simulink model "validation_simulations_elena_P"  (R2019b)
settings: Solver=FixedStepAuto  StartTime=0.0  StopTime=20  FixedStep=0.002  RelTol=1e-3
undefined symbols (not defined in the file or in its folder): Ao, Bo, Co, kalmf, Klqi_int, Klqi_state, Kpp_int, Kpp_state, Parameters
settings Model: Creator=Samsung  LastModifiedBy=pietr

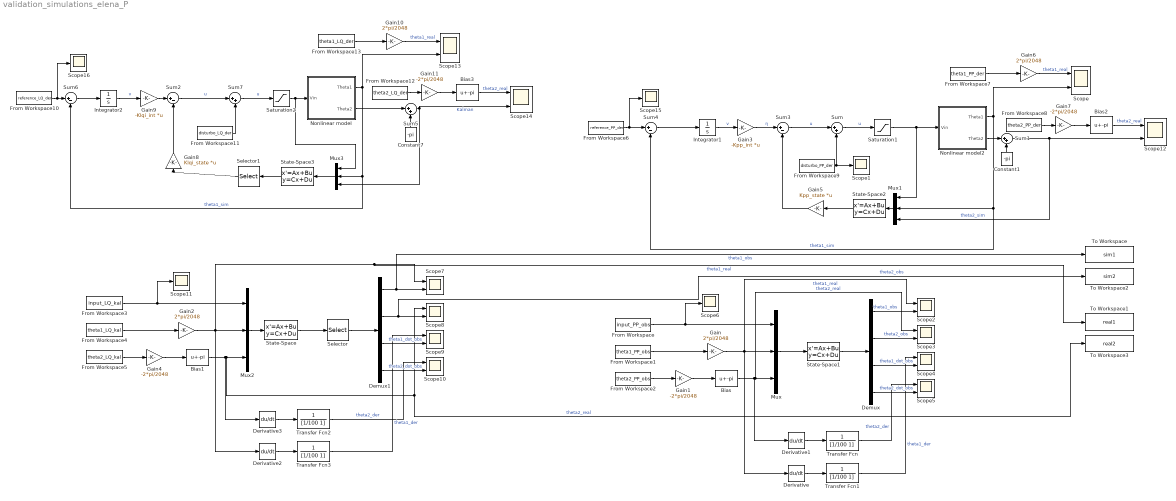
== system validation_simulations_elena_P ==
  Bias{,1..3} (4 alike) : Bias  Bias=-pi
  Constant1 : Constant  Value=-pi
  Constant7 : Constant  Value=-pi
  Demux : Demux
  Demux1 : Demux
  Derivative{,1..3} (4 alike) : Derivative
  From Workspace : FromWorkspace  VariableName=input_PP_obs  SampleTime=0
  From Workspace1 : FromWorkspace  VariableName=theta1_PP_obs  SampleTime=0
  From Workspace10 : FromWorkspace  VariableName=reference_LQ_der  SampleTime=0
  From Workspace11 : FromWorkspace  VariableName=disturbo_LQ_der  SampleTime=0
  From Workspace12 : FromWorkspace  VariableName=theta2_LQ_der  SampleTime=0
  From Workspace13 : FromWorkspace  VariableName=theta1_LQ_der  SampleTime=0
  From Workspace2 : FromWorkspace  VariableName=theta2_PP_obs  SampleTime=0
  From Workspace3 : FromWorkspace  VariableName=input_LQ_kal  SampleTime=0
  From Workspace4 : FromWorkspace  VariableName=theta1_LQ_kal  SampleTime=0
  From Workspace5 : FromWorkspace  VariableName=theta2_LQ_kal  SampleTime=0
  From Workspace6 : FromWorkspace  VariableName=reference_PP_der  SampleTime=0
  From Workspace7 : FromWorkspace  VariableName=theta1_PP_der  SampleTime=0
  From Workspace8 : FromWorkspace  VariableName=theta2_PP_der  SampleTime=0
  From Workspace9 : FromWorkspace  VariableName=disturbo_PP_der  SampleTime=0
  Gain{,2,6,10} (4 alike) : Gain  Gain=2*pi/2048
  Gain{1,4,7,11} (4 alike) : Gain  Gain=-2*pi/2048
  Gain3 : Gain  Gain=-Kpp_int  Multiplication=Matrix(K*u)
  Gain5 : Gain  Gain=Kpp_state  Multiplication=Matrix(K*u)
  Gain8 : Gain  Gain=Klqi_state  Multiplication=Matrix(K*u)
  Gain9 : Gain  Gain=-Klqi_int  Multiplication=Matrix(K*u)
  Integrator1 : Integrator
  Integrator2 : Integrator
  Mux{,1..3} (4 alike) : Mux  Inputs=3
  Nonlinear model : Subsystem
  Nonlinear model2 : Subsystem
  Saturation1 : Saturate  UpperLimit=10  LowerLimit=-10
  Saturation2 : Saturate  UpperLimit=10  LowerLimit=-10
  Scope{,2..5,7..10,12..14} (12 alike) : Scope  NumInputPorts=2
  Scope{1,6,11,15..16} (5 alike) : Scope
  Selector : Selector  InputPortWidth=6  IndexOptions=Index vector (dialog)  Indices=[3,4,5,6]  OutputSizes=1
  Selector1 : Selector  InputPortWidth=6  IndexOptions=Index vector (dialog)  Indices=[3,4,5,6]  OutputSizes=1
  State-Space : StateSpace  A=kalmf.A  B=kalmf.B  C=kalmf.C  D=kalmf.D  InitialCondition=[0,0,0,0]
  State-Space1 : StateSpace  A=Ao  B=Bo  C=Co  D=zeros(4,3)  InitialCondition=[0,0,0,0]
  State-Space2 : StateSpace  A=Ao  B=Bo  C=Co  D=zeros(4,3)  InitialCondition=[0,0,0,0]
  State-Space3 : StateSpace  A=kalmf.A  B=kalmf.B  C=kalmf.C  D=kalmf.D  InitialCondition=[0,0,0,0]
  Sum{,1,5,7} (4 alike) : Sum  Inputs=|++
  Sum{2..4,6} (4 alike) : Sum  Inputs=|+-
  To Workspace : ToWorkspace  VariableName=sim1  SampleTime=-1
      settings: Save2DSignal=2-D array (concatenate along first dimension)
  To Workspace1 : ToWorkspace  VariableName=real1  SampleTime=-1
      settings: Save2DSignal=2-D array (concatenate along first dimension)
  To Workspace2 : ToWorkspace  VariableName=sim2  SampleTime=-1
      settings: Save2DSignal=2-D array (concatenate along first dimension)
  To Workspace3 : ToWorkspace  VariableName=real2  SampleTime=-1
      settings: Save2DSignal=2-D array (concatenate along first dimension)
  Transfer Fcn{,1..3} (4 alike) : TransferFcn  Denominator=[1/100 1]
  wires:
  State-Space2/1 -> Gain5/1
  Sum4/1 -> Integrator1/1
  Nonlinear model2/2(Theta2) -> Sum1/1
  Gain5/1 -> Sum3/2
  Nonlinear model2/1(Theta1) -> Scope/2, Mux1/2, Sum4/2  "theta1_sim"
  Sum/1 -> Saturation1/1  "u"
  Constant1/1 -> Sum1/2
  Saturation1/1 -> Mux1/1, Nonlinear model2/1(Vin)
  Integrator1/1 -> Gain3/1  "v"
  Mux1/1 -> State-Space2/1
  Gain3/1 -> Sum3/1  "η"
  Sum1/1 -> Mux1/3, Scope12/2  "theta2_sim"
  Mux/1 -> State-Space1/1
  State-Space1/1 -> Demux/1
  Gain/1 -> Scope2/1, Derivative/1, Mux/2  "theta1_real"
  Gain1/1 -> Bias/1
  Demux/1 -> Scope2/2  "theta1_obs"
  Demux/2 -> Scope3/2  "theta2_obs"
  Demux/3 -> Scope4/2  "theta1_dot_obs"
  Demux/4 -> Scope5/2  "theta2_dot_obs"
  Derivative1/1 -> Transfer Fcn/1
  Derivative/1 -> Transfer Fcn1/1
  Transfer Fcn/1 -> Scope5/1  "theta2_der"
  Transfer Fcn1/1 -> Scope4/1  "theta1_der"
  From Workspace1/1 -> Gain/1
  From Workspace2/1 -> Gain1/1
  From Workspace/1 -> Scope6/1, Mux/1
  Bias/1 -> Scope3/1, Mux/3, Derivative1/1  "theta2_real"
  State-Space/1 -> Selector/1
  Mux2/1 -> State-Space/1
  From Workspace5/1 -> Gain4/1
  Transfer Fcn2/1 -> Scope10/1  "theta2_der"
  Demux1/1 -> To Workspace/1, Scope7/2  "theta1_obs"
  Bias1/1 -> Scope8/1, To Workspace3/1, Mux2/3, Derivative3/1  "theta2_real"
  From Workspace3/1 -> Scope11/1, Mux2/1
  Demux1/2 -> To Workspace2/1, Scope8/2  "theta2_obs"
  From Workspace4/1 -> Gain2/1
  Transfer Fcn3/1 -> Scope9/1  "theta1_der"
  Gain2/1 -> To Workspace1/1, Scope7/1, Derivative2/1, Mux2/2  "theta1_real"
  Demux1/4 -> Scope10/2  "theta2_dot_obs"
  Gain4/1 -> Bias1/1
  Demux1/3 -> Scope9/2  "theta1_dot_obs"
  Derivative3/1 -> Transfer Fcn2/1
  Derivative2/1 -> Transfer Fcn3/1
  Selector/1 -> Demux1/1
  From Workspace6/1 -> Scope15/1, Sum4/1
  From Workspace7/1 -> Gain6/1
  Gain6/1 -> Scope/1  "theta1_real"
  From Workspace8/1 -> Gain7/1
  Gain7/1 -> Bias2/1
  Bias2/1 -> Scope12/1  "theta2_real"
  Sum3/1 -> Sum/1  "u"
  From Workspace9/1 -> Sum/2, Scope1/1
  Sum7/1 -> Saturation2/1  "u"
  Saturation2/1 -> Mux3/1, Nonlinear model/1(Vin)
  Nonlinear model/2(Theta2) -> Sum5/1
  Gain9/1 -> Sum2/1
  State-Space3/1 -> Selector1/1
  Constant7/1 -> Sum5/2
  Mux3/1 -> State-Space3/1
  Selector1/1 -> Gain8/1
  Integrator2/1 -> Gain9/1  "v"
  Gain8/1 -> Sum2/2
  Sum6/1 -> Integrator2/1
  Sum5/1 -> Mux3/3, Scope14/2  "Kalman"
  From Workspace10/1 -> Scope16/1, Sum6/1
  Sum2/1 -> Sum7/1  "u"
  From Workspace11/1 -> Sum7/2
  From Workspace12/1 -> Gain11/1
  From Workspace13/1 -> Gain10/1
  Bias3/1 -> Scope14/1  "theta2_real"
  Nonlinear model/1(Theta1) -> Mux3/2, Sum6/2, Scope13/2  "theta1_sim"
  Gain10/1 -> Scope13/1  "theta1_real"
  Gain11/1 -> Bias3/1

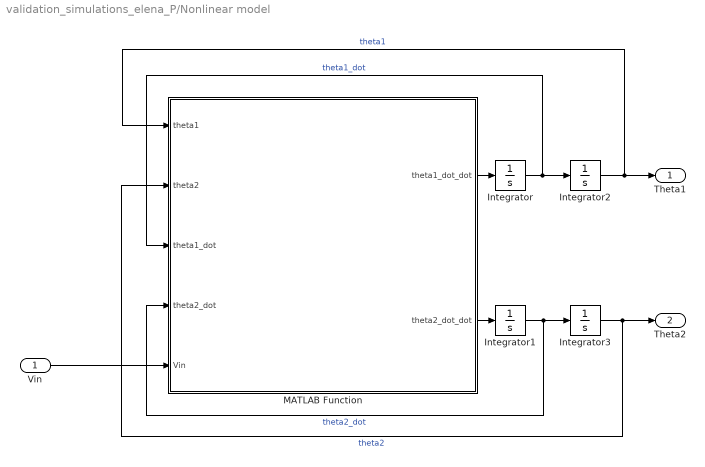
== system validation_simulations_elena_P/Nonlinear model ==
  Vin : Inport
  Integrator : Integrator  InitialCondition=0.05
  Integrator1 : Integrator  InitialCondition=0.05
  Integrator2 : Integrator
  Integrator3 : Integrator  InitialCondition=pi+0
  MATLAB Function : MATLAB Function  TreatAsAtomicUnit=on  mask{Pars=Parameters}
      mask prompts: Pars "Struct containing model parameters"
  Theta1 : Outport
  Theta2 : Outport  Port=2
  wires:
  Integrator/1 -> MATLAB Function/3(theta1_dot), Integrator2/1  "theta1_dot"
  Integrator1/1 -> MATLAB Function/4(theta2_dot), Integrator3/1  "theta2_dot"
  MATLAB Function/1(theta1_dot_dot) -> Integrator/1
  Integrator3/1 -> Theta2/1, MATLAB Function/2(theta2)  "theta2"
  MATLAB Function/2(theta2_dot_dot) -> Integrator1/1
  Integrator2/1 -> MATLAB Function/1(theta1), Theta1/1  "theta1"
  Vin/1 -> MATLAB Function/5(Vin)

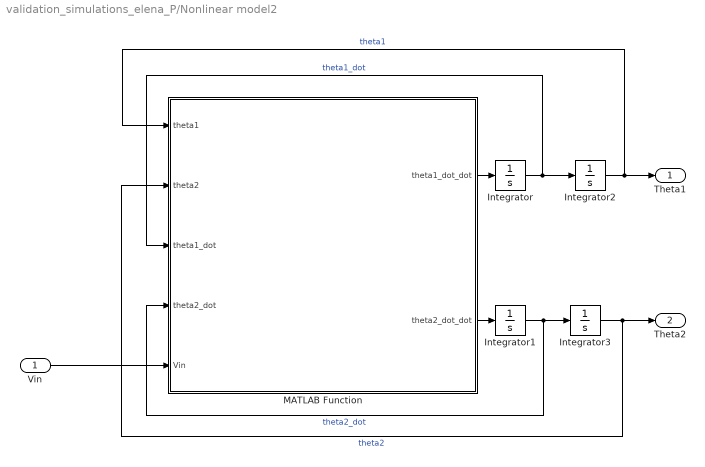
== system validation_simulations_elena_P/Nonlinear model2 ==
  Vin : Inport
  Integrator : Integrator  InitialCondition=0.05
  Integrator1 : Integrator  InitialCondition=0.05
  Integrator2 : Integrator  InitialCondition=0.1
  Integrator3 : Integrator  InitialCondition=pi+0.04
  MATLAB Function : MATLAB Function  TreatAsAtomicUnit=on  mask{Pars=Parameters}
      mask prompts: Pars "Struct containing model parameters"
  Theta1 : Outport
  Theta2 : Outport  Port=2
  wires:
  Integrator/1 -> MATLAB Function/3(theta1_dot), Integrator2/1  "theta1_dot"
  Integrator1/1 -> MATLAB Function/4(theta2_dot), Integrator3/1  "theta2_dot"
  MATLAB Function/1(theta1_dot_dot) -> Integrator/1
  Integrator3/1 -> Theta2/1, MATLAB Function/2(theta2)  "theta2"
  MATLAB Function/2(theta2_dot_dot) -> Integrator1/1
  Integrator2/1 -> MATLAB Function/1(theta1), Theta1/1  "theta1"
  Vin/1 -> MATLAB Function/5(Vin)

== matlab function validation_simulations_elena_P/Nonlinear model/MATLAB Function ==
  data: theta1 input; theta1_dot_dot output; theta2 input; theta1_dot input; theta2_dot input; Vin input; theta2_dot_dot output; Pars parameter
function [theta1_dot_dot,theta2_dot_dot] = fcn(theta1, theta2, theta1_dot, theta2_dot,Vin, Pars)

   k1 = Pars.Jeq + Pars.m2*(Pars.l1^2 + Pars.x2^2*sin(theta2)^2);
   k2 = Pars.m2*Pars.l1*Pars.x2*cos(theta2);
   k3 = 2*Pars.m2*Pars.x2^2*sin(theta2)*cos(theta2)*theta1_dot*theta2_dot - Pars.m2*Pars.l1*Pars.x2*sin(theta2)*theta2_dot^2 +Pars.Ks*theta1 - Pars.Km/Pars.Rm*Vin + (Pars.Km^2)/Pars.Rm*theta1_dot + Pars.Kf1*theta1_dot;
   k4 = Pars.m2*Pars.l1*Pars.x2*cos(theta2);
   k5 = Pars.m2*Pars.x2^2 + Pars.I2;
   k6 = - Pars.m2*Pars.x2^2*sin(theta2)*cos(theta2)*theta1_dot^2 + Pars.m2*Pars.g*Pars.x2*sin(theta2) + Pars.Kf2*theta2_dot;


theta1_dot_dot = (k2*k6 - k3*k5)/(k1*k5 - k2*k4);
theta2_dot_dot = -(k1*k6 - k3*k4)/(k1*k5 - k2*k4);

== matlab function validation_simulations_elena_P/Nonlinear model2/MATLAB Function ==
  data: theta1 input; theta1_dot_dot output; theta2 input; theta1_dot input; theta2_dot input; Vin input; theta2_dot_dot output; Pars parameter
function [theta1_dot_dot,theta2_dot_dot] = fcn(theta1, theta2, theta1_dot, theta2_dot,Vin, Pars)

   k1 = Pars.Jeq + Pars.m2*(Pars.l1^2 + Pars.x2^2*sin(theta2)^2);
   k2 = Pars.m2*Pars.l1*Pars.x2*cos(theta2);
   k3 = 2*Pars.m2*Pars.x2^2*sin(theta2)*cos(theta2)*theta1_dot*theta2_dot - Pars.m2*Pars.l1*Pars.x2*sin(theta2)*theta2_dot^2 +Pars.Ks*theta1 - Pars.Km/Pars.Rm*Vin + (Pars.Km^2)/Pars.Rm*theta1_dot + Pars.Kf1*theta1_dot;
   k4 = Pars.m2*Pars.l1*Pars.x2*cos(theta2);
   k5 = Pars.m2*Pars.x2^2 + Pars.I2;
   k6 = - Pars.m2*Pars.x2^2*sin(theta2)*cos(theta2)*theta1_dot^2 + Pars.m2*Pars.g*Pars.x2*sin(theta2) + Pars.Kf2*theta2_dot;


theta1_dot_dot = (k2*k6 - k3*k5)/(k1*k5 - k2*k4);
theta2_dot_dot = -(k1*k6 - k3*k4)/(k1*k5 - k2*k4);
